simulink model "tightening"  (R2023b)
settings: Solver=VariableStepAuto  StartTime=0.0  StopTime=10.0  RelTol=1e-3
settings Model: Creator=kailin  LastModifiedBy=kailin

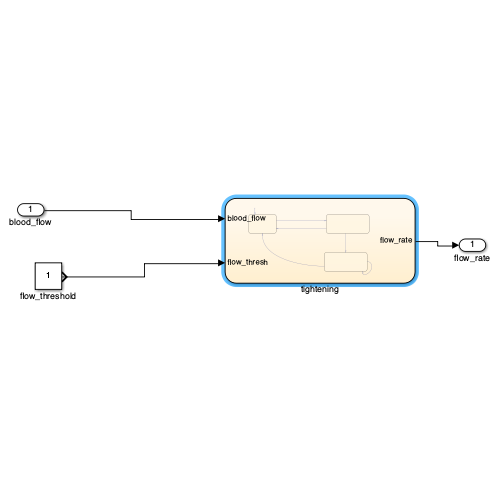
[thumbnail: Simulink's stored preview of the top-level diagram]
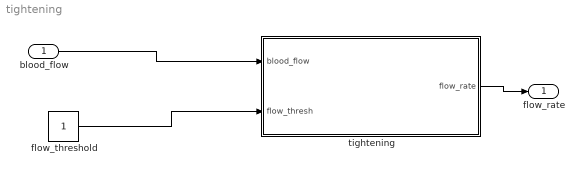
== system tightening ==
  blood_flow : Inport
  flow_threshold : Constant
  tightening : Stateflow chart  TreatAsAtomicUnit=on
  flow_rate : Outport
  wires:
  blood_flow/1 -> tightening/1(blood_flow)
  tightening/1(flow_rate) -> flow_rate/1
  flow_threshold/1 -> tightening/2(flow_thresh)

== stateflow chart tightening/tightening ==
  state Inflate
  state Hold
    entry:
    time_held = 0;
    during:
    time_held = time_held + t;
  state Deflate
    entry:
  (default) -> Inflate
  Inflate -> Hold : [blood_flow <= flow_thresh]
  Hold -> Inflate [order 1] : [blood_flow > flow_thresh]
  Deflate -> Inflate [order 1] : [blood_flow > 0]
  Hold -> Deflate [order 2] : [time_held >= hold_time]
  Deflate -> Deflate [order 2] : [blood_flow == 0]
  data: blood_flow input; flow_rate output; flow_thresh input
